simulink model "Model_3ac_2015a"  (R2015b)
settings: Solver=ode45  StartTime=0.0  StopTime=40  RelTol=1e-3
undefined symbols (not defined in the file): c1, c2, fhz, K1, K2, K3, Ts, wave
settings Model: Creator=s3blanch  LastModifiedBy=s3blanch
settings DataIOCC: SaveFormat=StructureWithTime
settings HardwareCC: ProdWordSize=32  ProdHWDeviceType=Specified

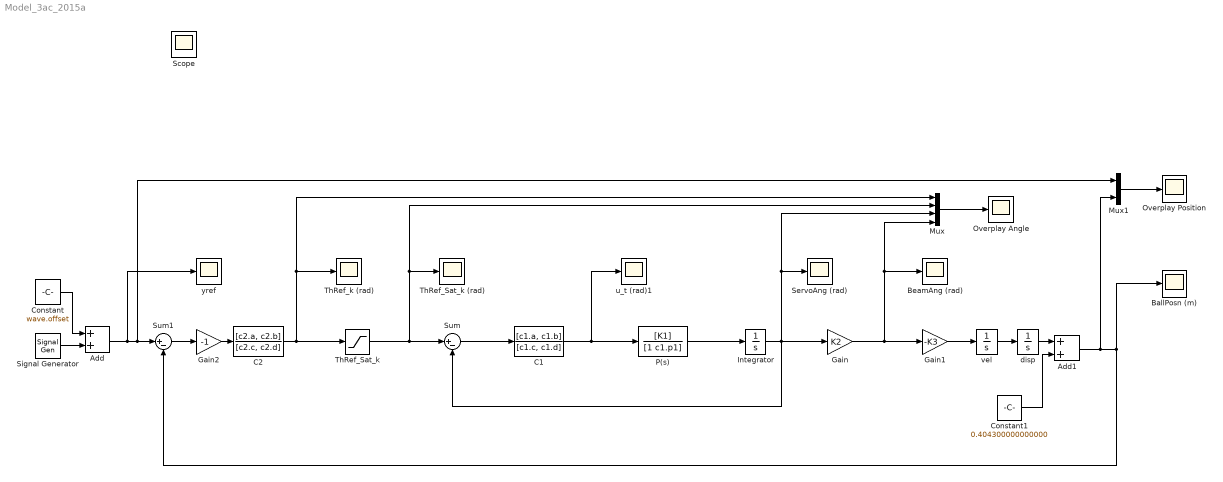
== system Model_3ac_2015a ==
  " BeamAng (rad)" : Scope
  Add : Sum
  Add1 : Sum
  BallPosn (m) : Scope
  C1 : DiscreteTransferFcn  Numerator=[c1.a, c1.b]  Denominator=[c1.c, c1.d]  SampleTime=Ts
  C2 : DiscreteTransferFcn  Numerator=[c2.a, c2.b]  Denominator=[c2.c, c2.d]  SampleTime=Ts
  Constant : Constant  Value=wave.offset
  Constant1 : Constant  Value=0.404300000000000
  Gain : Gain  Gain=K2
  Gain1 : Gain  Gain=-K3
  Gain2 : Gain  Gain=-1
  Integrator : Integrator
  Mux : Mux
  Mux1 : Mux  Inputs=2
  Overplay Angle : Scope
  Overplay Position : Scope
  P(s) : TransferFcn  Numerator=[K1]  Denominator=[1 c1.p1]
  ServoAng (rad) : Scope
  Signal Generator : SignalGenerator  WaveForm=square  Amplitude=-wave.amp  Frequency=fhz
  Sum : Sum  Inputs=|+-
  Sum1 : Sum  Inputs=|+-
  ThRef_Sat_k : Saturate  UpperLimit=0.7  LowerLimit=-0.7
  ThRef_Sat_k (rad) : Scope
  ThRef_k (rad) : Scope
  disp : Integrator
  u_t (rad)1 : Scope
  vel : Integrator
  yref : Scope
  Scope : Scope
  wires:
  P(s)/1 -> Integrator/1
  Integrator/1 -> Gain/1, Sum/2, Mux/3, ServoAng (rad)/1
  Mux/1 -> Overplay Angle/1
  Sum/1 -> C1/1
  C1/1 -> P(s)/1, u_t (rad)1/1
  Gain1/1 -> vel/1
  vel/1 -> disp/1
  C2/1 -> Mux/1, ThRef_k (rad)/1, ThRef_Sat_k/1
  Mux1/1 -> Overplay Position/1
  Signal Generator/1 -> Add/2
  Constant/1 -> Add/1
  Add/1 -> Mux1/1, Sum1/1, yref/1
  Gain/1 -> Gain1/1, " BeamAng (rad)"/1, Mux/4
  ThRef_Sat_k/1 -> Sum/1, Mux/2, ThRef_Sat_k (rad)/1
  disp/1 -> Add1/1
  Add1/1 -> Mux1/2, Sum1/2, BallPosn (m)/1
  Constant1/1 -> Add1/2
  Sum1/1 -> Gain2/1
  Gain2/1 -> C2/1
